simulink model "main"  (R2023b)
settings: Solver=VariableStepAuto  StartTime=0.0  StopTime=10  RelTol=1e-6
InitFcn:
  | test
libraries: truetime x2
settings Model: Creator=anton  LastModifiedBy=sunan
settings SolverCC: AlgebraicLoopSolver=TrustRegion
settings DataIOCC: ReturnWorkspaceOutputs=off
settings OptimizationCC: ReuseModelBlockBuffer=off
settings DebuggingCC: UnconnectedInputMsg=warning  UnconnectedOutputMsg=warning  UnconnectedLineMsg=warning  ArithmeticOperatorsInVariantConditions=warning
settings ModelReferenceCC: EnableRefExpFcnMdlSchedulingChecks=on
settings SFSimCC: SimUseLocalCustomCode=off  CustomCodeUndefinedFunction=UseInterfaceOnly
settings RTWCC: RTWUseLocalCustomCode=off  DLArmComputeVersion=19.05
settings CodeAppCC: StateflowObjectComments=on

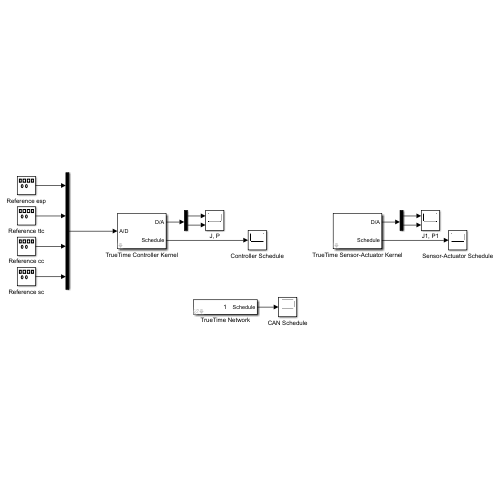
[thumbnail: Simulink's stored preview of the top-level diagram]
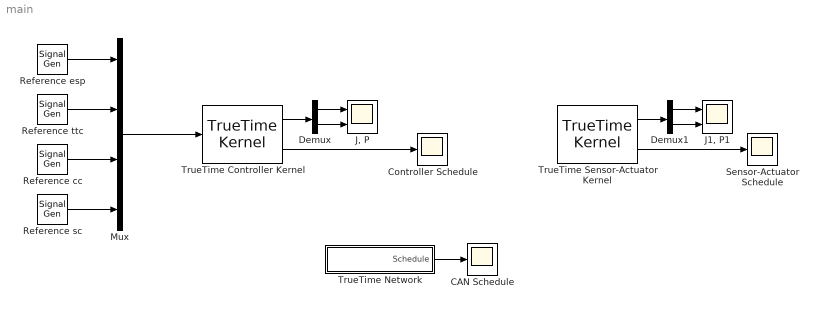
== system main ==
  CAN Schedule : Scope
  Controller Schedule : Scope
  Demux : Demux  Outputs=2
  Demux1 : Demux  Outputs=2
  "J, P" : Scope  NumInputPorts=2
  "J1, P1" : Scope  NumInputPorts=2
  Mux : Mux
  Reference cc : SignalGenerator  WaveForm=square  Amplitude=-1  Frequency=0.02
  Reference esp : SignalGenerator  WaveForm=square  Amplitude=-10  Frequency=0.02
  Reference sc : SignalGenerator  WaveForm=square  Amplitude=-1  Frequency=0.02
  Reference ttc : SignalGenerator  WaveForm=square  Amplitude=-1  Frequency=0.02
  Sensor-Actuator Schedule : Scope
  TrueTime Controller Kernel : truetime/TrueTime Kernel  sfun=control_sched_init  args=[]  ninputsoutputs=[4 2]  ntriggers=0  trigtype=falling  nwnodenbr=[]  clockoffsetdrift=[0 0]  schedoutput=on  battery=off  poweroutput=off
  TrueTime Network : Subsystem  AncestorBlock=truetime/TrueTime Network  mask(Real-Time Network){nwtype=CSMA/AMP (CAN), nwnbr=1, nnodes=2, rate=500000, minsize=80, lossprob=0, seed=0, bandwidths=[0.5 0.5], slotsize=512, schedule=[1 1 2], memsize=80000, buftype=Common buffer, overflow=Retransmit, dynSchedule=0, miniSlotSize=0, NIT=0, QSortMode=FIFO, sync=0, irtSchedule=0, nrtLength=0, nodeGraph=0, scheduleoutput=on}
      mask prompts: nwtype "Network type:"; nwnbr "Network number:"; nnodes "Number of nodes:"; rate "Data rate (bits/s):"; minsize "Minimum frame size (bits):"; lossprob "Loss probability (0-1):"; seed "Initial seed:"; bandwidths "Bandwidth allocations:"; slotsize "Slotsize (bits):"; schedule "Static schedule:"; memsize "Total switch memory (bits):"; buftype "Switch buffer type:"; overflow "Switch overflow behavior:"; dynSchedule "Dynamic Schedule:"; miniSlotSize "Mini slot size (bits):"; NIT "Network idle time (bits):"; QSortMode "Input Queue Sorted by:"; sync "Synchronization length (bits):"; irtSchedule "IRT Schedule [msgID from to start arrival]:"; nrtLength "RT Class 1/NRT length (bits):"; nodeGraph "Node connection graph (nbrOfnodes x nbrOfNodes):"; scheduleoutput "Show Schedule output port:"
      mask init:
      | ttnetwork_callback(gcb,nwnbr,nnodes,scheduleoutput)
      mask TypeOptions nwtype: CSMA/CD (Ethernet) | CSMA/AMP (CAN) | Round Robin | FDMA | TDMA | Switched Ethernet | FlexRay | PROFINET | NCM
      mask Callback nwtype: ttnetwork_callback
      mask TypeOptions buftype: Common buffer | Symmetric output buffers
      mask TypeOptions overflow: Retransmit | Drop
      mask TypeOptions QSortMode: FIFO | Priority
      mask Display: disp(nwnbr)
  TrueTime Sensor-Actuator Kernel : truetime/TrueTime Kernel  sfun=sensact_sched_init  args=[]  ninputsoutputs=[0 2]  ntriggers=0  trigtype=falling  nwnodenbr=[]  clockoffsetdrift=[0 0]  schedoutput=on  battery=off  poweroutput=off
  wires:
  TrueTime Controller Kernel/2 -> Controller Schedule/1
  Demux/2 -> "J, P"/2
  TrueTime Controller Kernel/1 -> Demux/1
  Demux/1 -> "J, P"/1
  TrueTime Network/1(Schedule) -> CAN Schedule/1
  TrueTime Sensor-Actuator Kernel/1 -> Demux1/1
  Demux1/1 -> "J1, P1"/1
  Demux1/2 -> "J1, P1"/2
  TrueTime Sensor-Actuator Kernel/2 -> Sensor-Actuator Schedule/1
  Mux/1 -> TrueTime Controller Kernel/1
  Reference esp/1 -> Mux/1
  Reference ttc/1 -> Mux/2
  Reference sc/1 -> Mux/4
  Reference cc/1 -> Mux/3

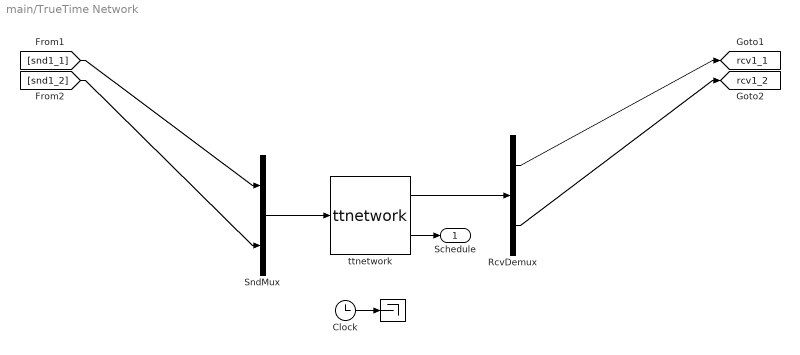
== system main/TrueTime Network ==
  " " : Terminator
  Clock : Clock
  RcvDemux : Demux  Outputs=2
      settings: DisplayOption=none
  SndMux : Mux  Inputs=2
  ttnetwork : S-Function  FunctionName=ttnetwork  Parameters=nwtype,nwnbr,nnodes,rate,minsize,lossprob,bandwidths,slotsize,schedule,memsize,buftype,overflow,seed,dynSchedule,miniSlotSize,NIT,QSortMode,sync,irtSchedule,nrtLength,nodeGraph  SFunctionDeploymentMode=off  EnableBusSupport=off
  Schedule : Outport
  tag scope: rcv1_1=global, rcv1_2=global
  wires:
  Clock/1 -> " "/1
  SndMux/1 -> ttnetwork/1
  ttnetwork/1 -> RcvDemux/1
  ttnetwork/2 -> Schedule/1
  [snd1_1] -> SndMux/1
  [snd1_2] -> SndMux/2
  RcvDemux/1 -> [rcv1_1]
  RcvDemux/2 -> [rcv1_2]
